simulink model "Simple_TDMA"  (Simulink 9.0)
settings: Solver=VariableStepAuto  StartTime=0.0  StopTime=10/fs  RelTol=1e-3  EnableMultiTasking=on
undefined symbols (not defined in the file): fs, gray
libraries: commdigbbndam3 x3, visionsources x2, commutil2 x2
settings Model: SuppressorTable=22 serialization::archive 11 0 6 0 0 0 0 0  Creator=15337  LastModifiedBy=changgang
settings DataIOCC: LimitDataPoints=on  SaveFormat=Dataset
settings DebuggingCC: UnderspecifiedInitializationDetection=Simplified  MergeDetectMultiDrivingBlocksExec=error  AllowSymbolicDim=off
settings HardwareCC: ProdBitPerPointer=64  ProdBitPerSizeT=64  ProdBitPerPtrDiffT=64  ProdLargestAtomicFloat=Float  ProdIntDivRoundTo=Zero  ProdEndianess=LittleEndian  ProdWordSize=64  ProdHWDeviceType=Intel->x86-64 (Windows64)

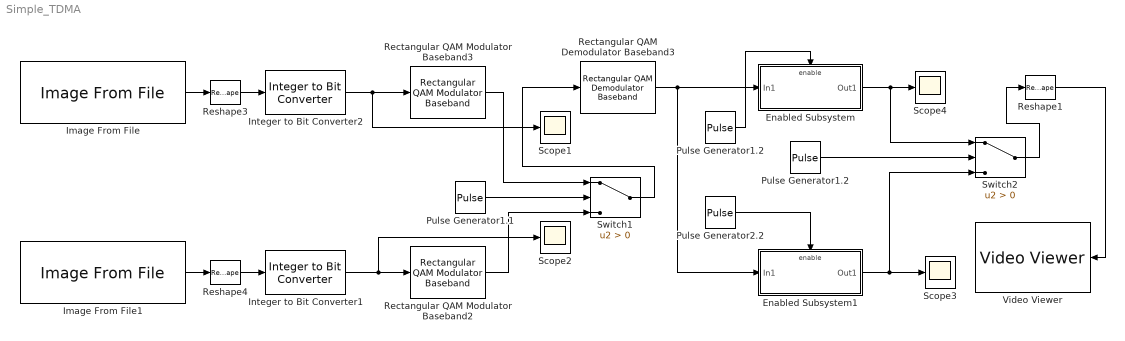
== system Simple_TDMA ==
  Enabled Subsystem : Subsystem  TreatAsAtomicUnit=on
  Enabled Subsystem1 : Subsystem  TreatAsAtomicUnit=on
  Image From File : visionsources/Image From File  Tag=vipblks_nd  FileName=/Users/changgang/Documents/Changgang Zheng/Bachelor/Final Year 19-20/Winter Semester/Wireless and Optical Transmission Systems/Assignments/Matlab Code for Assignment/Figure/Asuka_2_value.png  imagePorts=One multidimensional signal  Ts=1/fs  ImageDataType=double  Signed=on  WordLength=16  sdImageDataType=uint(8)  FractionLengthMode=User-defined  FractionLength=15  OutPortLabels=G
      settings: SourceProductName=Computer Vision System Toolbox
  Image From File1 : visionsources/Image From File  Tag=vipblks_nd  FileName=/Users/changgang/Documents/Changgang Zheng/Bachelor/Final Year 19-20/Winter Semester/Wireless and Optical Transmission Systems/Assignments/Matlab Code for Assignment/Figure/Asuka_2_value.png  imagePorts=One multidimensional signal  Ts=1/fs  ImageDataType=double  Signed=on  WordLength=16  sdImageDataType=uint(8)  FractionLengthMode=User-defined  FractionLength=15  OutPortLabels=G
      settings: SourceProductName=Computer Vision System Toolbox
  Integer to Bit Converter1 : commutil2/Integer to Bit Converter  nbits=1  signedInputValues=Unsigned  bitOrder=LSB first  outDtype=boolean
  Integer to Bit Converter2 : commutil2/Integer to Bit Converter  nbits=1  signedInputValues=Unsigned  bitOrder=LSB first  outDtype=boolean
  Pulse Generator1.1 : DiscretePulseGenerator  PulseType=Time based  Period=0.1  PulseWidth=50
  Pulse Generator1.2 : DiscretePulseGenerator  PulseType=Time based  Period=0.1  PulseWidth=50
  "Pulse Generator1.2 " : DiscretePulseGenerator  PulseType=Time based  Period=0.1  PulseWidth=50
  Pulse Generator2.2 : DiscretePulseGenerator  PulseType=Time based  Period=0.1  PulseWidth=50  PhaseDelay=0.05
  Rectangular QAM Demodulator Baseband3 : commdigbbndam3/Rectangular QAM Demodulator Baseband  M=16  OutType=Bit  DecType=Hard decision  VarSource=Dialog  Variance=1  Dec=Gray  Mapping=[0:15]  PowType=Min. distance between symbols  MinDist=2  AvgPow=1  PeakPow=1  Ph=0  outDtype1=Inherit via internal rule  outDtype2=Inherit via internal rule  derotateFactorWordLen=16  derotateFactorDataTypeStr=Inherit: Same word length as input  derotateFactorLastDataTypeStr=Inherit: Same word length as input  denormFactorWordLen=16  denormFactorDataTypeStr=Inherit: Same word length as input  denormFactorLastDataTypeStr=Inherit: Same word length as input  prodOutWordLen=32  prodOutOverflowMode=Wrap  prodOutRoundingMode=Floor  prodOutOvFlMode=off  prodOutOvFlModeLastStrValue=off  sumWordLen=32
  Rectangular QAM Modulator Baseband2 : commdigbbndam3/Rectangular QAM Modulator Baseband  M=16  InType=Bit  Enc=Gray  Mapping=[0:15]  PowType=Min. distance between symbols  MinDist=2  AvgPow=1  PeakPow=1  Ph=0  outDtype=double  outWordLen=16  outUDDataType=sfix(16)  outFracLenMode=Best precision  outFracLen=15  outDataTypeStr=double  outLastDataTypeStr=double
  Rectangular QAM Modulator Baseband3 : commdigbbndam3/Rectangular QAM Modulator Baseband  M=16  InType=Bit  Enc=Gray  Mapping=[0:15]  PowType=Min. distance between symbols  MinDist=2  AvgPow=1  PeakPow=1  Ph=0  outDtype=double  outWordLen=16  outUDDataType=sfix(16)  outFracLenMode=Best precision  outFracLen=15  outDataTypeStr=double  outLastDataTypeStr=double
  Reshape1 : Reshape  OutputDimensionality=Customize  OutputDimensions=[1050,700]
  Reshape3 : Reshape
  Reshape4 : Reshape
  Scope{1..4} (4 alike) : Scope
  Switch1 : Switch  Criteria=u2 > Threshold
  Switch2 : Switch  Criteria=u2 > Threshold
  Video Viewer : VideoViewer  colormapValue=gray(256)  FigPos=[416 742 775 458]
  wires:
  Pulse Generator1.1/1 -> Switch1/2
  "Pulse Generator1.2 "/1 -> Enabled Subsystem/Enable
  Pulse Generator2.2/1 -> Enabled Subsystem1/Enable
  Switch1/1 -> Rectangular QAM Demodulator Baseband3/1
  Integer to Bit Converter1/1 -> Scope2/1, Rectangular QAM Modulator Baseband2/1
  Rectangular QAM Modulator Baseband3/1 -> Switch1/1
  Rectangular QAM Modulator Baseband2/1 -> Switch1/3
  Rectangular QAM Demodulator Baseband3/1 -> Enabled Subsystem/1(In1), Enabled Subsystem1/1(In1)
  Reshape1/1 -> Video Viewer/1
  Enabled Subsystem/1(Out1) -> Switch2/1, Scope4/1
  Enabled Subsystem1/1(Out1) -> Scope3/1, Switch2/3
  Pulse Generator1.2/1 -> Switch2/2
  Integer to Bit Converter2/1 -> Scope1/1, Rectangular QAM Modulator Baseband3/1
  Image From File1/1 -> Reshape4/1
  Image From File/1 -> Reshape3/1
  Reshape3/1 -> Integer to Bit Converter2/1
  Reshape4/1 -> Integer to Bit Converter1/1
  Switch2/1 -> Reshape1/1

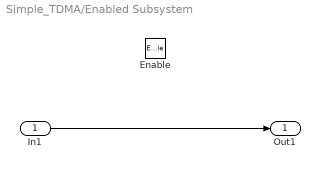
== system Simple_TDMA/Enabled Subsystem ==
  In1 : Inport
  Enable : EnablePort
  Out1 : Outport
  wires:
  In1/1 -> Out1/1

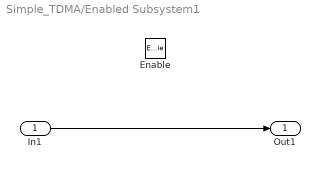
== system Simple_TDMA/Enabled Subsystem1 ==
  In1 : Inport
  Enable : EnablePort
  Out1 : Outport
  wires:
  In1/1 -> Out1/1
